simulink model "motor_control_FOC_SVM"  (Simulink 7.9)
settings: Solver=ode45  StartTime=0.0  StopTime=10.0  RelTol=1e-3
libraries: powerlib x10, c28xdmclib x1
settings Model: Creator=Dmitriy  LastModifiedBy=Dmitriy
settings RTWCC: GenerateMakefile=off

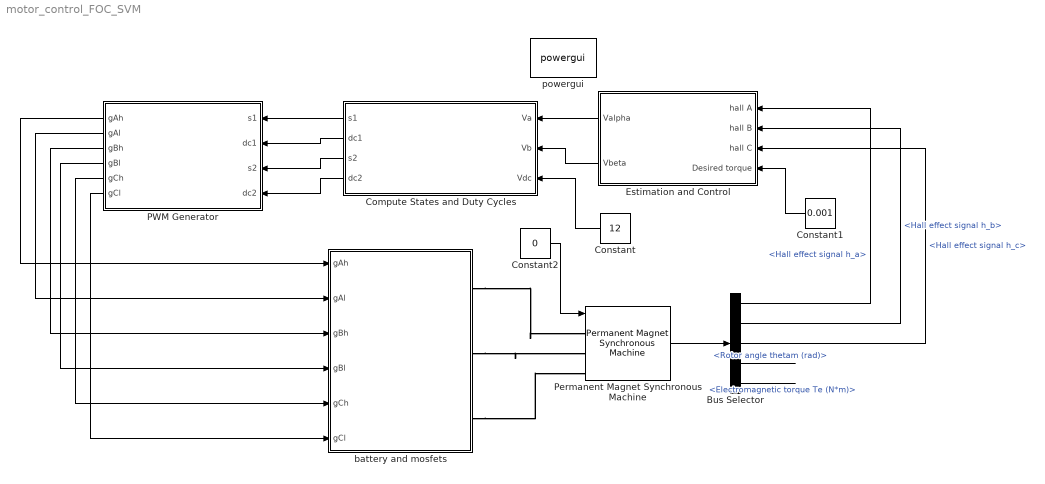
== system motor_control_FOC_SVM ==
  Bus Selector : BusSelector  OutputSignals=Hall effect signal h_a,Hall effect signal h_b,Hall effect signal h_c,Rotor angle thetam (rad),Electromagnetic torque Te (N*m)
  Compute States and Duty Cycles : MATLAB Function  TreatAsAtomicUnit=on
  Constant : Constant  Value=12
  Constant1 : Constant  Value=0.001
  Constant2 : Constant  Value=0
  Estimation and Control : Subsystem
  PWM Generator : MATLAB Function  TreatAsAtomicUnit=on  SystemSampleTime=10^-7
  Permanent Magnet Synchronous Machine : powerlib/Machines/Permanent Magnet Synchronous Machine  NbPhases=3  FluxDistribution=Sinusoidal  RotorType=Round  MechanicalLoad=Torque Tm  PresetModel=No  ShowDetailedParameters=on  Resistance=28.2  Inductance=8.5e-3  dqInductances=[0.006365 0.006365]  La=1940*10^-6  MachineConstant=Torque Constant (N.m / A_peak)  Flux=0.0060333  VoltageCst=2.1887  TorqueCst=18.1*10^-3  Flat=120  Mechanical=[0.0001 5.396e-005 2 0]  PolePairs=2  InitialConditions=[0,0, 0,0]  InitialConditions5ph=[0 0 0 0 0 0]  TsPowergui=0  TsBlock=-1  RefAngle=Aligned with phase A axis (original Park)
  battery and mosfets : Subsystem
  powergui : powerlib/powergui  Priority=1  SimulationMode=Continuous  SolverType=Tustin  SampleTime=50e-6  frequency=60  SPID=off  DisableSnubberDevices=off  DisableRonSwitches=off  DisableVfSwitches=off  SwTol=0  Interpol=off  DisplayEquations=off  FunctionMessages=off  frequencyindice=0  Pbase=100e6  ErrMax=1e-4  Iterations=50  UnitsV=kV  UnitsW=MW  echomessages=off  HookPort=off  EnableUseOfTLC=off  x0status=blocks  RestoreLinks=warning  ResistiveCurrentMeasurement=off  Ylog=off  Xlog=on  ShowGrid=off  save=off  variable=ZData  ZoomFFT=off  StartTime=0.0  cycles=1  DisplayStyle=1  FreqAxis=off  MaxFrequency=1000  frequencyindicesteady=1  display=off  methode=off
  wires:
  Permanent Magnet Synchronous Machine/1 -> Bus Selector/1
  Bus Selector/1 -> Estimation and Control/1(hall A)  "<Hall effect signal h_a>"
  Bus Selector/3 -> Estimation and Control/3(hall C)  "<Hall effect signal h_c>"
  Bus Selector/4 -> ?  "<Rotor angle thetam (rad)>"
  Bus Selector/5 -> ?  "<Electromagnetic torque Te (N*m)>"
  Bus Selector/2 -> Estimation and Control/2(hall B)  "<Hall effect signal h_b>"
  Estimation and Control/1(Valpha) -> Compute States and Duty Cycles/1(Va)
  Estimation and Control/2(Vbeta) -> Compute States and Duty Cycles/2(Vb)
  Compute States and Duty Cycles/1(s1) -> PWM Generator/1(s1)
  Compute States and Duty Cycles/2(dc1) -> PWM Generator/2(dc1)
  Compute States and Duty Cycles/3(s2) -> PWM Generator/3(s2)
  Compute States and Duty Cycles/4(dc2) -> PWM Generator/4(dc2)
  PWM Generator/6(gCl) -> battery and mosfets/6(gCl)
  PWM Generator/5(gCh) -> battery and mosfets/5(gCh)
  PWM Generator/4(gBl) -> battery and mosfets/4(gBl)
  PWM Generator/3(gBh) -> battery and mosfets/3(gBh)
  PWM Generator/2(gAl) -> battery and mosfets/2(gAl)
  PWM Generator/1(gAh) -> battery and mosfets/1(gAh)
  Constant/1 -> Compute States and Duty Cycles/3(Vdc)
  Constant1/1 -> Estimation and Control/4(Desired torque)
  Constant2/1 -> Permanent Magnet Synchronous Machine/1
  connections:
  battery and mosfets/RConn1 -- Permanent Magnet Synchronous Machine/LConn1
  battery and mosfets/RConn2 -- Permanent Magnet Synchronous Machine/LConn2
  battery and mosfets/RConn3 -- Permanent Magnet Synchronous Machine/LConn3

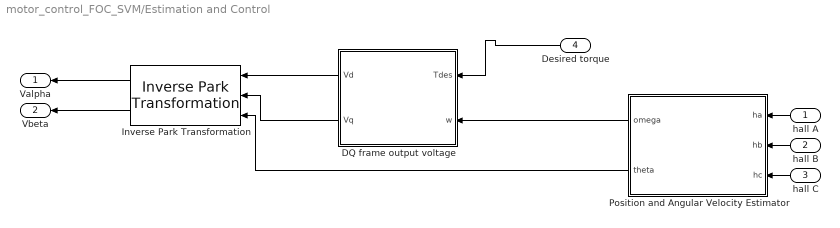
== system motor_control_FOC_SVM/Estimation and Control ==
  hall A : Inport
  hall B : Inport  Port=2
  hall C : Inport  Port=3
  Desired torque : Inport  Port=4
  DQ frame output voltage : MATLAB Function  TreatAsAtomicUnit=on
  Inverse Park Transformation : c28xdmclib/Inverse Park Transformation
  Position and Angular Velocity Estimator : MATLAB Function  TreatAsAtomicUnit=on
  Valpha : Outport
  Vbeta : Outport  Port=2
  wires:
  Position and Angular Velocity Estimator/1(omega) -> DQ frame output voltage/2(w)
  Desired torque/1 -> DQ frame output voltage/1(Tdes)
  hall A/1 -> Position and Angular Velocity Estimator/1(ha)
  hall B/1 -> Position and Angular Velocity Estimator/2(hb)
  hall C/1 -> Position and Angular Velocity Estimator/3(hc)
  Position and Angular Velocity Estimator/2(theta) -> Inverse Park Transformation/3
  DQ frame output voltage/2(Vq) -> Inverse Park Transformation/2
  DQ frame output voltage/1(Vd) -> Inverse Park Transformation/1
  Inverse Park Transformation/1 -> Valpha/1
  Inverse Park Transformation/2 -> Vbeta/1

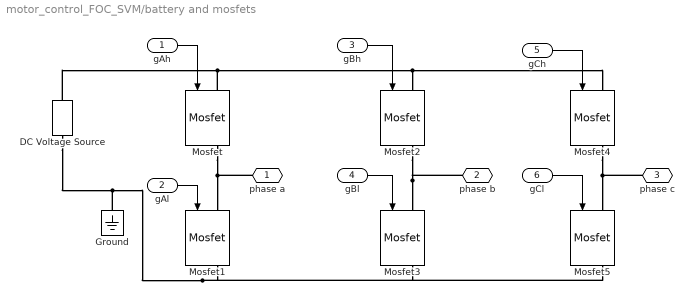
== system motor_control_FOC_SVM/battery and mosfets ==
  gAh : Inport
  gAl : Inport  Port=2
  gBh : Inport  Port=3
  gBl : Inport  Port=4
  gCh : Inport  Port=5
  gCl : Inport  Port=6
  DC Voltage Source : powerlib/Electrical Sources/DC Voltage Source  Amplitude=12  Measurements=None
  Ground : powerlib/Elements/Ground  LConnTagsString=a
  Mosfet{,1..5} (6 alike) : powerlib/Power Electronics/Mosfet  Ron=0.1  Lon=0  Rd=0.01  Vfd=0  IC=0  Rs=1e5  Cs=inf  Measurements=on
  phase a : PMIOPort  Port=1  Side=Right
  phase b : PMIOPort  Port=2  Side=Right
  phase c : PMIOPort  Port=3  Side=Right
  wires:
  gCl/1 -> Mosfet5/1
  gCh/1 -> Mosfet4/1
  gBh/1 -> Mosfet2/1
  gBl/1 -> Mosfet3/1
  gAl/1 -> Mosfet1/1
  gAh/1 -> Mosfet/1
  connections:
  Mosfet/RConn1 -- Mosfet1/LConn1 -- phase a/RConn1
  Mosfet2/RConn1 -- Mosfet3/LConn1 -- phase b/RConn1
  phase c/RConn1 -- Mosfet4/RConn1 -- Mosfet5/LConn1
  Ground/LConn1 -- Mosfet3/RConn1 -- Mosfet5/RConn1 -- Mosfet1/RConn1 -- DC Voltage Source/LConn1
  Mosfet/LConn1 -- Mosfet2/LConn1 -- Mosfet4/LConn1 -- DC Voltage Source/RConn1

== matlab function Estimation and Control/DQ frame output voltage ==
  data: Tdes input double; Vd output double; w input double; Vq output double
function [Vd,Vq] = computeDQOutput(Tdes,w)
%#codegen
%take the desired torque current 
% speed and compute the output voltage vector in the DQ
%frame. 

L = 1940*10^-6;
R = 28.2;
Ke = (1.895*10^-3)*9.54929659643; % convert to V/(rad/s) 
Kt = 1.81*10^3; %Nm/Amp

%because I is assumed to be on Q axis, T = KtI
Ides = Tdes/Kt;

%bemf is on q axis
bemf = Ke*w;

%inductor impedance 
ZL = L*w;

Vq = bemf+Ides*R;
Vd = -ZL*Ides;

== matlab function Estimation and Control/Position and Angular Velocity Estimator ==
  data: omega output double; ha input double; theta output double; hb input double; hc input double
function [omega,theta] = rotor_est(ha,hb,hc)
%#codegen
%estimate the position of the rotor in degrees electrical
Test = .001;

persistent prev_t;
persistent t;
persistent prev_halls;
persistent w;
persistent theta1;

if(isempty(prev_t))
    prev_t=0;
    t = 0;
    prev_halls = [ha hb hc];
    w = 0;
    theta1 = getThetaFromHalls([ha hb hc]);
end

t = t+Test;
halls = [ha hb hc];

if(sum(halls == prev_halls)==3)
    theta1 = theta1 + w*Test;
    return;
else
    w = getOmegaFromHalls(halls,prev_halls,t,prev_t);
    if(w>0)
        theta1=getThetaFromHalls(halls);
    else
        theta1 = getThetaFromHalls(prev_halls);
    end
    prev_t = t;
    prev_halls = halls;
end

theta = theta1;
omega = wrapTo2Pi(w);

end

== matlab function Compute States and Duty Cycles ==
  data: Va input double; s1 output double; dc1 output double; Vb input double; s2 output double; Vdc input double; dc2 output double
function [s1,dc1, s2, dc2] = statesAndCycles(Va,Vb, Vdc)
%#codegen

%Given desired Valpha and Vbeta, and the supply voltage, compute the inverter states to toggle
%between and the duty cycle of each

%right now we're saying that the length of each state vector is Vdc, which
%is probably wrong

ang = wrapTo2Pi(angle(Va+1i*Vb));

sext = floor(ang/(pi/3));

%states as defined in james mevey's thesis
%v1, v2 are complex values of the voltages
switch sext
    case 0
        s1 = 1;
        v1 = Vdc;
        
        s2 = 2;
        temp = pol2cart(Vdc, pi/3);
        v2 = temp(1)+i*temp(2);
        
    case 1
        s1 = 2;
        temp = pol2cart(Vdc, pi/3);
        v1 = temp(1)+1i*temp(2);
        
        s2 = 3;
        temp = pol2cart(Vdc, 2*pi/3);
        v2 = temp(1)+1i*temp(2);
        
    case 2
        s1 = 3;
        temp = pol2cart(Vdc, 2*pi/3);
        v1 = temp(1)+1i*temp(2);
        
        s2 = 4;
        temp = pol2cart(Vdc, pi);
        v2 = temp(1)+1i*temp(2);
    case 3
        s1 = 4;
        temp = pol2cart(Vdc, pi);
        v1 = temp(1)+1i*temp(2);
        
        s2 = 5;
        temp = pol2cart(Vdc, 4*pi/3);
        v2 = temp(1)+1i*temp(2);
    case 4 
        s1 = 5;
        temp = pol2cart(Vdc, 4*pi/3);
        v1 = temp(1)+1i*temp(2);
        
        
        s2 = 6;
        temp = pol2cart(Vdc, 5*pi/3);
        v2 = temp(1)+1i*temp(2);
    case 5
        s1 = 6;
        temp = pol2cart(Vdc, 5*pi/3);
        v1 = temp(1)+1i*temp(2);
        
        s2 = 1;
        v2 = Vdc
end

%solve for intersection of v1 line and v2 line translated to the desired
%place

num = Va-imag(v2)*Vb/real(v2)- imag(v1);
den = real(v1) - imag(v2)/real(v2);

xint = num/den;
yint = (imag(v1)/real(v1))*xint;

%duty cycle 1 equals length of sv1 divided by Vdc, which is nominal length
dc1 = sqrt(xint^2+yint^2)/Vdc;

%duty cycle 2 is distance from the tip of sv1 to the desired point, divided
%by Vdc

dc2 = sqrt((xint-Va)^2 +(yint - Vb)^2)/Vdc;

== matlab function PWM Generator ==
  data: s1 input double; gAh output double; dc1 input double; s2 input double; dc2 input double; gAl output double; gBh output double; gBl output double; gCh output double; gCl output double
function [gAh,gAl,gBh,gBl,gCh,gCl] = generateGateSignals(s1,dc1,s2,dc2)
%#codegen
Tsamp = 10^-7;
Tswitch = 10^-4;



persistent k;

if(isempty(k))
    k=1;
end

if(k > 1000)
    k=1;
end

%determine the current output
if(k<1000*dc1)
    output = s1;
else
    if(k>1000-1000*dc2)
        output = s2;
    else
        output = 0;
    end
end

%generate the gate signals
switch output
    case 0
        gates = [0 1 0 1 0 1];
        
    case 1
        gates = [1 0 0 1 0 1];
        
    case 2
        gates = [1 0 1 0 0 1];
        
    case 3
        gates = [0 1 1 0 0 1];
        
    case 4
        gates = [0 1 1 0 1 0];
        
    case 5
        gates = [0 1 0 1 0 0];
    
    case 6
        gates = [1 0 0 1 1 0];
end

gAh = gates(1);
gAl = gates(2);
gBh = gates(3);
gBl = gates(4);
gCh = gates(5);
gCl = gates(6);

k=k+1;
